simulink model "segway_torque_control"  (R2022a)
settings: Solver=FixedStepAuto  StartTime=0.0  StopTime=10  FixedStep=1e-3  RelTol=1e-3
PreLoadFcn:
  | preload
InitFcn:
  | init
  | preload
values from neighbouring files (symbols this model uses):
  A1 = [0 0   1 0 ... (first row only)    [plant.m]
  A2 = [0   1 ... (first row only)    [plant.m]
  alpha = n * Kt    [plant.m]
  B1 = [0 0 ... (first row only)    [plant.m]
  B2 = [0    0 ... (first row only)    [plant.m]
  C1 = [1 0 0 0 ... (first row only)    [plant.m]
  C2 = [1 0 ... (first row only)    [plant.m]
  chi0 = zeros(N_ukf, 2*N_ukf+1)    [UKF_params.m]
  D = 0.2    [params.m]
  D1 = zeros(4, 2)    [plant.m]
  D2 = zeros(2)    [plant.m]
  Fd = sysd.A    [LKF_params.m]
  fm = evalin('base', 'fm')    [f.m]    (also in params.m = 0.0022)
  fw = 0.0    (= 0)    [params.m]
  g = 9.81    [params.m]
  Gd = sysd.B    [LKF_params.m]
  h = 0.39    [params.m]
  H_ekf = [0 1 0 0 0 0 0 ... (first row only)    [EKF_params.m]
  H_lkf = [0 1 0 0 0 0 0 ... (first row only)    [LKF_params.m]
  H_ukf = [0 1 0 0 0 0 0 ... (first row only)    [UKF_params.m]
  Jm = 1e-5    (= 1e-05)    [params.m]
  Jphi = M * (W^2 + D^2) / 12    (= 0.126774333333)    [params.m]
  Jpsi = M * L^2 / 3    (= 0.08910525)    [params.m]
  Jw = m * R^2 / 2    (= 0.01146068)    [params.m]
  Jwx = m * (3*R^2 + hw^2) / 12    (= 0.00610456)    [params.m]
  K_lqr = lqrd(s4.A, s4.B, QQ, RR, Ts)    [control.m]
  Kt = 2.28    [params.m]
  L = h / 2    (= 0.195)    [params.m]
  lambda_ukf = alpha_ukf^2 * (N_ukf + kappa_ukf) - N_ukf    [UKF_params.m]
  M = 7.03    [params.m]
  m = 1.54    [params.m]
  n = 1    [params.m]
  N_ukf = length(x0_ukf)    [UKF_params.m]
  P0_ekf = eye(7)*0.1    [EKF_params.m]
  P0_lkf = eye(7)*0.1    [LKF_params.m]
  P0_ukf = eye(7)*0.1    [UKF_params.m]
  Q_ekf = [0.1*Ts^4/4     Ts^3/2     0          Ts^2/2     0          0          0 ... (first row only)    [EKF_params.m]
  Q_lkf = [Ts^4/4     Ts^3/2     0          Ts^2/2     0          0          0 ... (first row only)    [LKF_params.m]
  Q_ukf = [0.0025*Ts^4 Ts^3/2     0          Ts^2/2     0          0          0 ... (first row only)    [UKF_params.m]
  R = 0.122    [params.m]
  R_ekf = [sigma_y_ekf(1) 0          0          0          0 ... (first row only)    [EKF_params.m]
  R_lkf = [sigma_y(1) 0          0          0          0 ... (first row only)    [LKF_params.m]
  R_ukf = [sigma_y_ukf(1) 0          0          0          0 ... (first row only)    [UKF_params.m]
  Ts = 0.01    [params.m]
  W = 0.42    [params.m]
  w_c_ukf = diag(wi*ones([1, 2*N_ukf+1]))    [UKF_params.m]
  w_m_ukf = wi*ones([1, 2*N_ukf+1])    [UKF_params.m]
  x0_ekf = [0; 0; 0; 0; 0; 0; 0]    [EKF_params.m]
  x0_lkf = [0; 0; 0; 0; 0; 0; 0]    [LKF_params.m]
  x0_ukf = [0; 0; 0; 0; 0; 0; 0]    [UKF_params.m]
  Z0_ukf = zeros(5, 2*N_ukf+1)    [UKF_params.m]
undefined symbols (not defined in the file or in its folder): X, Y, Z
libraries: sm_lib x18, nesl_utility x14, simulink_extras x4, simulink x1
(part 1 of 2)
settings Model: Creator=skakd  LastModifiedBy=Yoggi
settings SolverCC: ZeroCrossControl=EnableAll  ZeroCrossAlgorithm=Adaptive  EnableFixedStepZeroCrossing=on

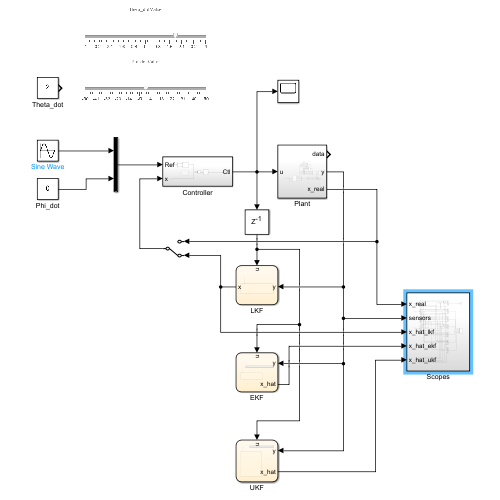
[thumbnail: Simulink's stored preview of the top-level diagram]
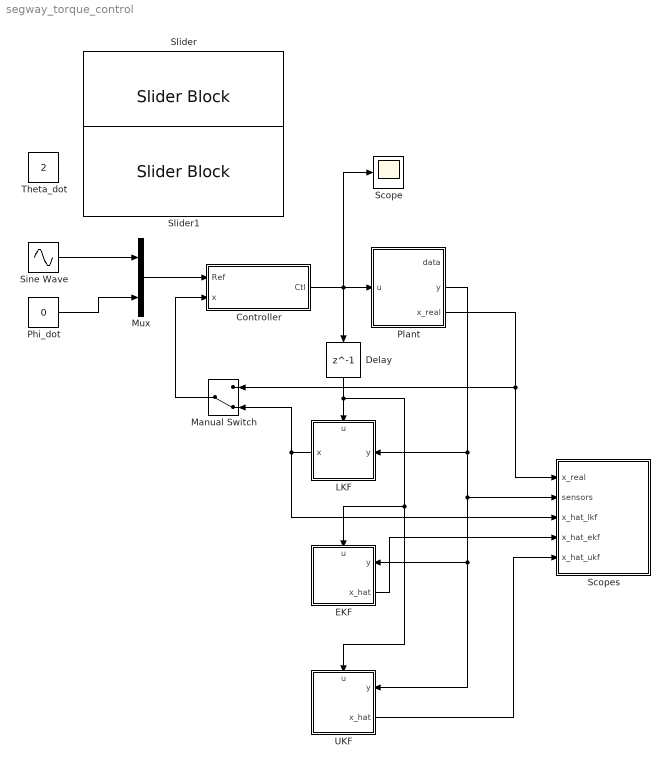
== system segway_torque_control ==
  Controller : Subsystem  SystemSampleTime=0.01
  Delay : Delay  DelayLength=1
  EKF : Stateflow chart  TreatAsAtomicUnit=on  SystemSampleTime=Ts
      settings: PortSchema="{\"entries\":[{\"content\":{\"sides\":[{\"content\":{\"connectorIds\":[]},\"type\":\"ConnectorPlacement.EquallySpacedRectSide\",\"uuid\":\"7365e1c5-a084-40ff-bf9b-f6bb3324d08a\"},{\"content\":{\"connectorIds\":[\"In2\",\"Out1\"],\"side\":\"RIGHT\"},\"type\":\"ConnectorPlacement.EquallySpacedRectSide\",\"uuid\":\"e745d55e-2f97-4317-b982-3a71d81393c6\"},{\"content\":{\"connectorIds\":[\"In1\"],\"side\":\"TOP\"},\"type\":\"ConnectorPlacement.EquallySpacedRectSide\",\"uuid\":\"33cc398c-7f08-41ce-89d7-3873ba12ad1e\"}]},\"type\":\"ConnectorPlacement.EquallySpacedConnector\",\"uuid\":\"9c830667-db1c-4875-b9da-b2b8107bc2bd\"}],\"packageUris\":[\"http://schema.mathworks.com/mf0/Connector/R2020b\"],\"version\":\"1.0\"}"
  LKF : Stateflow chart  TreatAsAtomicUnit=on  SystemSampleTime=Ts
      settings: PortSchema="{\"entries\":[{\"content\":{\"sides\":[{\"content\":{\"connectorIds\":[\"Out1\"]},\"type\":\"ConnectorPlacement.EquallySpacedRectSide\",\"uuid\":\"7365e1c5-a084-40ff-bf9b-f6bb3324d08a\"},{\"content\":{\"connectorIds\":[\"In2\"],\"side\":\"RIGHT\"},\"type\":\"ConnectorPlacement.EquallySpacedRectSide\",\"uuid\":\"e745d55e-2f97-4317-b982-3a71d81393c6\"},{\"content\":{\"connectorIds\":[\"In1\"],\"side\":\"TOP\"},\"type\":\"ConnectorPlacement.EquallySpacedRectSide\",\"uuid\":\"33cc398c-7f08-41ce-89d7-3873ba12ad1e\"}]},\"type\":\"ConnectorPlacement.EquallySpacedConnector\",\"uuid\":\"9c830667-db1c-4875-b9da-b2b8107bc2bd\"}],\"packageUris\":[\"http://schema.mathworks.com/mf0/Connector/R2020b\"],\"version\":\"1.0\"}"
  Manual Switch : ManualSwitch  CurrentSetting=0
  Mux : Mux  Inputs=2
  Phi_dot : Constant  Value=0
  Plant : Subsystem
  Scope : Scope
  Scopes : Subsystem
  Sine Wave : Sin  SampleTime=0
  Slider : SliderBlock  ScaleMin=-4  ScaleMax=4
  Slider1 : SliderBlock  ScaleMin=-50  ScaleMax=50
  Theta_dot : Constant  Value=2
  UKF : Stateflow chart  TreatAsAtomicUnit=on  SystemSampleTime=Ts
      settings: PortSchema="{\"entries\":[{\"content\":{\"sides\":[{\"content\":{\"connectorIds\":[]},\"type\":\"ConnectorPlacement.EquallySpacedRectSide\",\"uuid\":\"7365e1c5-a084-40ff-bf9b-f6bb3324d08a\"},{\"content\":{\"connectorIds\":[\"In2\",\"Out1\"],\"side\":\"RIGHT\"},\"type\":\"ConnectorPlacement.EquallySpacedRectSide\",\"uuid\":\"e745d55e-2f97-4317-b982-3a71d81393c6\"},{\"content\":{\"connectorIds\":[\"In1\"],\"side\":\"TOP\"},\"type\":\"ConnectorPlacement.EquallySpacedRectSide\",\"uuid\":\"33cc398c-7f08-41ce-89d7-3873ba12ad1e\"}]},\"type\":\"ConnectorPlacement.EquallySpacedConnector\",\"uuid\":\"9c830667-db1c-4875-b9da-b2b8107bc2bd\"}],\"packageUris\":[\"http://schema.mathworks.com/mf0/Connector/R2020b\"],\"version\":\"1.0\"}"
  wires:
  Phi_dot/1 -> Mux/2
  Mux/1 -> Controller/1(Ref)
  Controller/1(Ctl) -> Plant/1(u), Scope/1, Delay/1
  Plant/2(y) -> UKF/2(y), EKF/2(y), Scopes/2(sensors), LKF/2(y)
  Plant/3(x_real) -> Manual Switch/1, Scopes/1(x_real)
  Delay/1 -> EKF/1(u), UKF/1(u), LKF/1(u)
  LKF/1(x) -> Scopes/3(x_hat_lkf), Manual Switch/2
  Manual Switch/1 -> Controller/2(x)
  EKF/1(x_hat) -> Scopes/4(x_hat_ekf)
  Sine Wave/1 -> Mux/1
  UKF/1(x_hat) -> Scopes/5(x_hat_ukf)

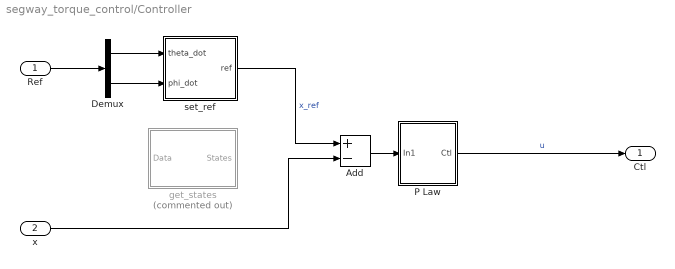
== system segway_torque_control/Controller ==
  Ref : Inport
  x : Inport  Port=2
  Add : Sum  Inputs=+-
  Demux : Demux  Outputs=2
  P Law : Subsystem  TreatAsAtomicUnit=on  SystemSampleTime=0.01
  get_states : Subsystem  Commented=on
  set_ref : Subsystem
  Ctl : Outport  VectorParamsAs1DForOutWhenUnconnected=off
  wires:
  P Law/1(Ctl) -> Ctl/1  "u"
  set_ref/1(ref) -> Add/1  "x_ref"
  Ref/1 -> Demux/1
  Demux/1 -> set_ref/1(theta_dot)
  Demux/2 -> set_ref/2(phi_dot)
  Add/1 -> P Law/1(In1)
  x/1 -> Add/2

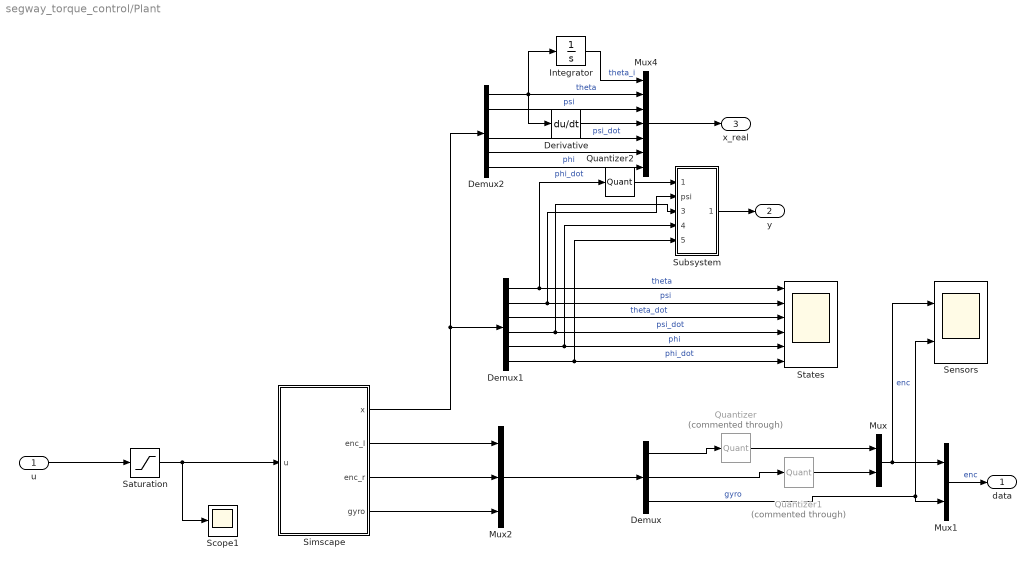
== system segway_torque_control/Plant ==
  u : Inport
  Demux : Demux  Outputs=3
  Demux1 : Demux  Outputs=6
  Demux2 : Demux  Outputs=6
  Derivative : Derivative
  Integrator : Integrator
  Mux : Mux  Inputs=2
  Mux1 : Mux  Inputs=2
  Mux2 : Mux  Inputs=3
  Mux4 : Mux  Inputs=7
  Quantizer : Quantizer  Commented=through  QuantizationInterval=pi/45
  Quantizer1 : Quantizer  Commented=through  QuantizationInterval=pi/45
  Quantizer2 : Quantizer  QuantizationInterval=pi/45
  Saturation : Saturate  UpperLimit=40  LowerLimit=-40
  Scope1 : Scope
  Sensors : Scope  NumInputPorts=2
  Simscape : Subsystem  Variant=on  VariantControl=Choice
  States : Scope  NumInputPorts=6
  Subsystem : Subsystem  TreatAsAtomicUnit=on  SystemSampleTime=Ts
  data : Outport
  y : Outport  Port=2
  x_real : Outport  Port=3
  wires:
  Mux2/1 -> Demux/1
  Demux/1 -> Quantizer/1
  Demux/2 -> Quantizer1/1
  Mux/1 -> Mux1/1, Sensors/1  "enc"
  Demux/3 -> Mux1/2, Sensors/2  "gyro"
  Demux1/3 -> States/3  "theta_dot"
  Demux1/1 -> States/1, Quantizer2/1  "theta"
  Demux1/4 -> Subsystem/3(psi_dot), States/4  "psi_dot"
  Demux1/6 -> Subsystem/5(phi_dot), States/6  "phi_dot"
  Demux1/2 -> Subsystem/2(psi), States/2  "psi"
  Demux1/5 -> Subsystem/4(phi), States/5  "phi"
  u/1 -> Saturation/1
  Saturation/1 -> Scope1/1, Simscape/1(u)
  Simscape/1(x) -> Demux2/1, Demux1/1
  Simscape/2(enc_l) -> Mux2/1
  Simscape/3(enc_r) -> Mux2/2
  Simscape/4(gyro) -> Mux2/3
  Mux1/1 -> data/1  "enc"
  Quantizer/1 -> Mux/1
  Quantizer1/1 -> Mux/2
  Demux2/1 -> Derivative/1, Mux4/2, Integrator/1  "theta"
  Integrator/1 -> Mux4/1  "theta_i"
  Demux2/2 -> Mux4/3  "psi"
  Demux2/4 -> Mux4/5  "psi_dot"
  Demux2/5 -> Mux4/6  "phi"
  Demux2/6 -> Mux4/7  "phi_dot"
  Mux4/1 -> x_real/1
  Derivative/1 -> Mux4/4
  Quantizer2/1 -> Subsystem/1(In1)
  Subsystem/1(Out1) -> y/1

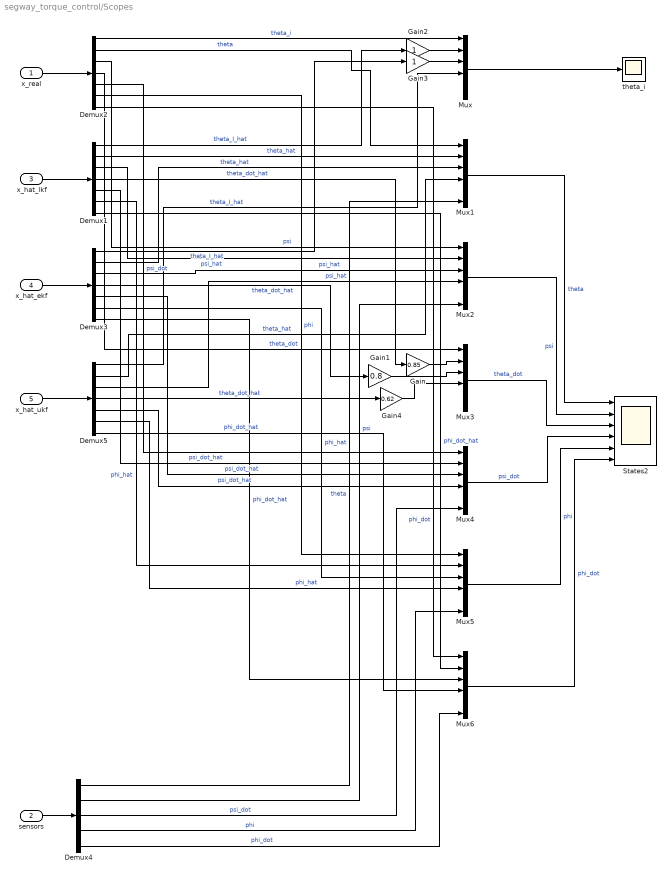
== system segway_torque_control/Scopes ==
  x_real : Inport
  sensors : Inport  Port=2
  x_hat_lkf : Inport  Port=3
  x_hat_ekf : Inport  Port=4
  x_hat_ukf : Inport  Port=5
  Demux{1..3,5} (4 alike) : Demux  Outputs=7
  Demux4 : Demux  Outputs=5
  Gain : Gain  Gain=0.85
  Gain1 : Gain  Gain=0.8
  Gain2 : Gain
  Gain3 : Gain
  Gain4 : Gain  Gain=0.62
  Mux{,1..6} (7 alike) : Mux  Inputs=6
  States2 : Scope  NumInputPorts=6
  theta_i : Scope
  wires:
  x_hat_lkf/1 -> Demux1/1
  x_real/1 -> Demux2/1
  Demux2/1 -> Mux/1  "theta_i"
  Demux1/1 -> Gain2/1  "theta_I_hat"
  Demux2/2 -> Mux1/1  "theta"
  Demux1/2 -> Mux1/2  "theta_hat"
  Demux2/3 -> Mux2/1  "psi"
  Demux2/4 -> Mux3/1  "theta_dot"
  Demux2/5 -> Mux4/1  "psi_dot"
  Demux2/6 -> Mux5/1  "phi"
  Demux2/7 -> Mux6/1  "phi_dot"
  Demux1/3 -> Mux2/2  "psi_hat"
  Demux1/4 -> Gain/1  "theta_dot_hat"
  Demux1/5 -> Mux4/2  "psi_dot_hat"
  Demux1/6 -> Mux5/2  "phi_hat"
  Demux1/7 -> Mux6/2  "phi_dot_hat"
  Mux1/1 -> States2/1  "theta"
  Mux2/1 -> States2/2  "psi"
  Mux3/1 -> States2/3  "theta_dot"
  Mux4/1 -> States2/4  "psi_dot"
  Mux5/1 -> States2/5  "phi"
  Mux6/1 -> States2/6  "phi_dot"
  Gain/1 -> Mux3/2
  x_hat_ekf/1 -> Demux3/1
  Mux/1 -> theta_i/1
  Demux3/1 -> Gain3/1  "theta_I_hat"
  Demux3/2 -> Mux1/3  "theta_hat"
  Demux3/3 -> Mux2/3  "psi_hat"
  Demux3/4 -> Gain1/1  "theta_dot_hat"
  Demux3/5 -> Mux4/3  "psi_dot_hat"
  Demux3/6 -> Mux5/3  "phi_hat"
  Demux3/7 -> Mux6/3  "phi_dot_hat"
  Gain1/1 -> Mux3/3
  Gain2/1 -> Mux/2
  Gain3/1 -> Mux/3
  sensors/1 -> Demux4/1
  Demux4/1 -> Mux1/6  "theta"
  Demux4/2 -> Mux2/6  "psi"
  Demux4/3 -> Mux4/6  "psi_dot"
  Demux4/4 -> Mux5/6  "phi"
  Demux4/5 -> Mux6/6  "phi_dot"
  x_hat_ukf/1 -> Demux5/1
  Demux5/1 -> Mux/4  "theta_I_hat"
  Demux5/2 -> Mux1/4  "theta_hat"
  Demux5/3 -> Mux2/4  "psi_hat"
  Demux5/4 -> Gain4/1  "theta_dot_hat"
  Demux5/5 -> Mux4/4  "psi_dot_hat"
  Demux5/6 -> Mux5/4  "phi_hat"
  Demux5/7 -> Mux6/4  "phi_dot_hat"
  Gain4/1 -> Mux3/4

== system segway_torque_control/Controller/P Law ==
  In1 : Inport
  Gain : Gain  Gain=K_lqr  Multiplication=Matrix(K*u)
  Ctl : Outport
  wires:
  Gain/1 -> Ctl/1
  In1/1 -> Gain/1

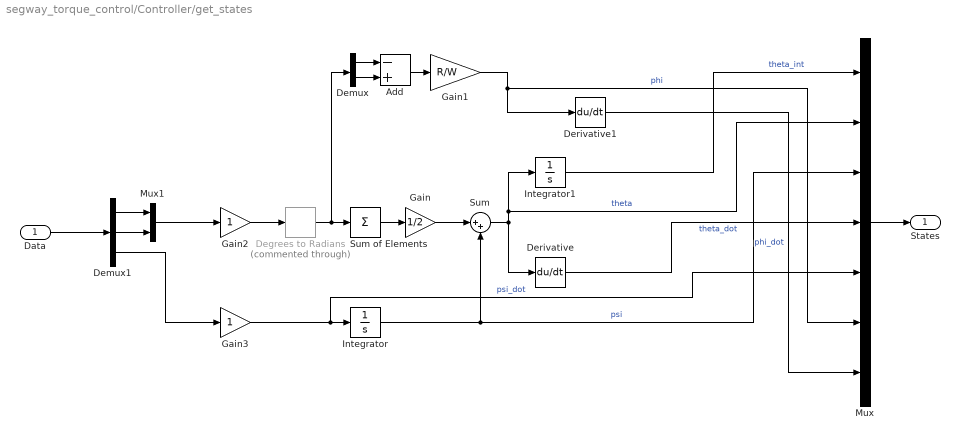
== system segway_torque_control/Controller/get_states ==
  Data : Inport
  Add : Sum  Inputs=-+
  Degrees to Radians : simulink_extras/Transformations/Degrees to Radians  Commented=through
  Demux : Demux  Outputs=2
  Demux1 : Demux  Outputs=3
  Derivative : Derivative
  Derivative1 : Derivative  CoefficientInTFapproximation=0.01
  Gain : Gain  Gain=1/2
  Gain1 : Gain  Gain=R/W
  Gain2 : Gain
  Gain3 : Gain
  Integrator : Integrator
  Integrator1 : Integrator
  Mux : Mux  Inputs=7
  Mux1 : Mux  Inputs=2
  Sum : Sum  Inputs=|++
  Sum of Elements : Sum  Inputs=+
  States : Outport  VectorParamsAs1DForOutWhenUnconnected=off
  wires:
  Gain/1 -> Sum/1
  Degrees to Radians/1 -> Demux/1, Sum of Elements/1
  Integrator/1 -> Sum/2, Mux/3  "psi"
  Data/1 -> Demux1/1
  Mux1/1 -> Gain2/1
  Sum/1 -> Mux/2, Integrator1/1, Derivative/1  "theta"
  Derivative/1 -> Mux/4  "theta_dot"
  Sum of Elements/1 -> Gain/1
  Gain3/1 -> Mux/5, Integrator/1  "psi_dot"
  Integrator1/1 -> Mux/1  "theta_int"
  Demux/1 -> Add/1
  Demux/2 -> Add/2
  Add/1 -> Gain1/1
  Gain1/1 -> Mux/6, Derivative1/1  "phi"
  Derivative1/1 -> Mux/7  "phi_dot"
  Mux/1 -> States/1
  Demux1/1 -> Mux1/1
  Demux1/2 -> Mux1/2
  Demux1/3 -> Gain3/1
  Gain2/1 -> Degrees to Radians/1

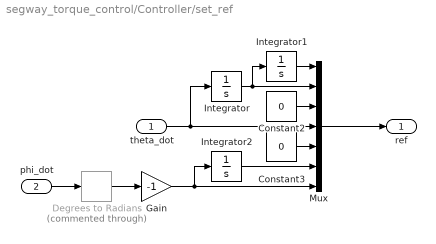
== system segway_torque_control/Controller/set_ref ==
  theta_dot : Inport
  phi_dot : Inport  Port=2
  Constant2 : Constant  Value=0
  Constant3 : Constant  Value=0
  Degrees to Radians : simulink_extras/Transformations/Degrees to Radians  Commented=through
  Gain : Gain  Gain=-1
  Integrator : Integrator
  Integrator1 : Integrator
  Integrator2 : Integrator
  Mux : Mux  Inputs=7
  ref : Outport  VectorParamsAs1DForOutWhenUnconnected=off
  wires:
  Constant2/1 -> Mux/3
  Constant3/1 -> Mux/5
  Mux/1 -> ref/1
  Integrator/1 -> Integrator1/1, Mux/2
  phi_dot/1 -> Degrees to Radians/1
  Integrator2/1 -> Mux/6
  Integrator1/1 -> Mux/1
  theta_dot/1 -> Integrator/1, Mux/4
  Degrees to Radians/1 -> Gain/1
  Gain/1 -> Integrator2/1, Mux/7

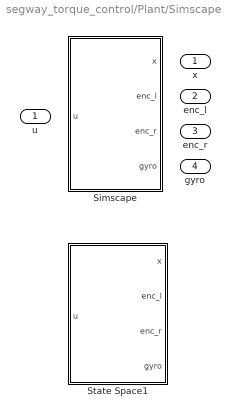
== system segway_torque_control/Plant/Simscape ==
  u : Inport
  Simscape : Subsystem  VariantControl=(default)
  State Space1 : Subsystem  VariantControl=is_simscape == 0
  x : Outport
  enc_l : Outport  Port=2
  enc_r : Outport  Port=3
  gyro : Outport  Port=4

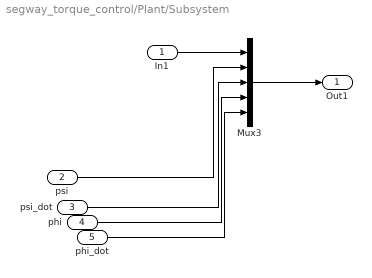
== system segway_torque_control/Plant/Subsystem ==
  In1 : Inport
  psi : Inport  Port=2
  psi_dot : Inport  Port=3
  phi : Inport  Port=4
  phi_dot : Inport  Port=5
  Mux3 : Mux  Inputs=5
  Out1 : Outport
  wires:
  In1/1 -> Mux3/1
  phi_dot/1 -> Mux3/5
  phi/1 -> Mux3/4
  Mux3/1 -> Out1/1
  psi_dot/1 -> Mux3/3
  psi/1 -> Mux3/2

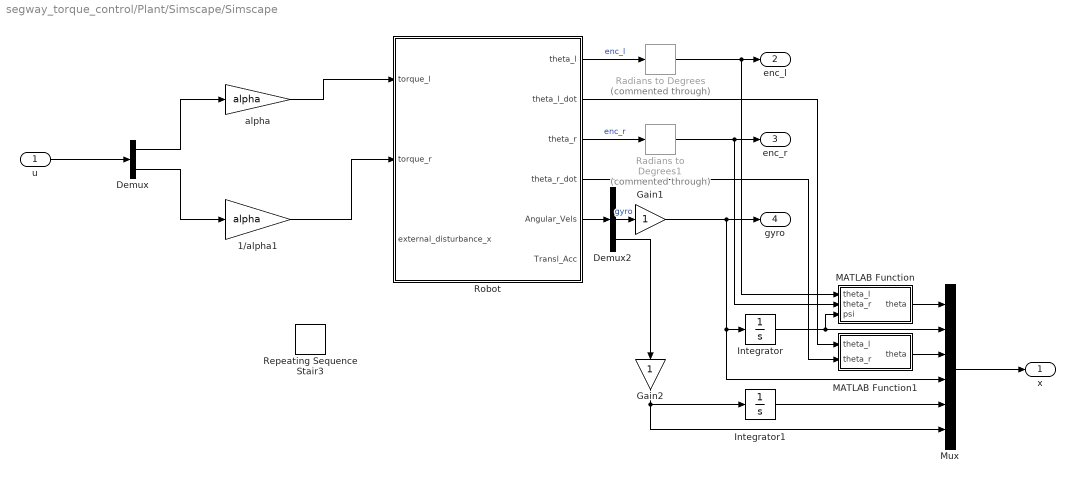
== system segway_torque_control/Plant/Simscape/Simscape ==
  u : Inport
  1/alpha1 : Gain  Gain=alpha
  Demux : Demux  Outputs=2
  Demux2 : Demux  Outputs=3
  Gain1 : Gain
  Gain2 : Gain
  Integrator : Integrator
  Integrator1 : Integrator
  MATLAB Function : MATLAB Function  TreatAsAtomicUnit=on
  MATLAB Function1 : MATLAB Function  TreatAsAtomicUnit=on
  Mux : Mux  Inputs=6
  Radians to Degrees : simulink_extras/Transformations/Radians to Degrees  Commented=through
  Radians to Degrees1 : simulink_extras/Transformations/Radians to Degrees  Commented=through
  Repeating Sequence Stair3 : simulink/Sources/Repeating Sequence Stair  OutValues=[0 0 0 0 0 0 0 0 0 0 0 0 15 0 0 0 0 0 0 0 0 0 0 0 0 0 0 0 0 0 0 0 0 0 0 0 0 0 0 0].'  tsamp=0.1  OutMin=[]  OutMax=[]  OutDataTypeStr=double  OutputDataTypeScalingMode=double  OutDataType=fixdt(0,8)  ConRadixGroup=Best Precision: Vector-wise  OutScaling=2^-12
  Robot : Subsystem
  alpha : Gain  Gain=alpha
  x : Outport
  enc_l : Outport  Port=2
  enc_r : Outport  Port=3
  gyro : Outport  Port=4
  wires:
  Robot/5(Angular_Vels) -> Demux2/1
  Demux2/2 -> Gain1/1  "gyro"
  Radians to Degrees1/1 -> MATLAB Function/2(theta_r), enc_r/1
  Robot/3(theta_r) -> Radians to Degrees1/1  "enc_r"
  Radians to Degrees/1 -> MATLAB Function/1(theta_l), enc_l/1
  Robot/1(theta_l) -> Radians to Degrees/1  "enc_l"
  Gain1/1 -> gyro/1, Mux/4, Integrator/1
  u/1 -> Demux/1
  Mux/1 -> x/1
  Integrator/1 -> MATLAB Function/3(psi), Mux/2
  Integrator1/1 -> Mux/5
  MATLAB Function/1(theta) -> Mux/1
  MATLAB Function1/1(theta) -> Mux/3
  Robot/2(theta_l_dot) -> MATLAB Function1/1(theta_l)
  Robot/4(theta_r_dot) -> MATLAB Function1/2(theta_r)
  Gain2/1 -> Integrator1/1, Mux/6
  Demux2/3 -> Gain2/1
  alpha/1 -> Robot/1(torque_l)
  1/alpha1/1 -> Robot/2(torque_r)
  Demux/1 -> alpha/1
  Demux/2 -> 1/alpha1/1

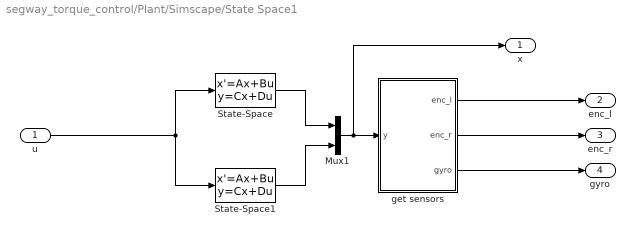
== system segway_torque_control/Plant/Simscape/State Space1 ==
  u : Inport
  Mux1 : Mux  Inputs=2
  State-Space : StateSpace  A=A1  B=B1  C=C1  D=D1  InitialCondition=0
  State-Space1 : StateSpace  A=A2  B=B2  C=C2  D=D2  InitialCondition=0
  get sensors : MATLAB Function  TreatAsAtomicUnit=on
  x : Outport
  enc_l : Outport  Port=2
  enc_r : Outport  Port=3
  gyro : Outport  Port=4
  wires:
  get sensors/3(gyro) -> gyro/1
  get sensors/2(enc_r) -> enc_r/1
  State-Space1/1 -> Mux1/2
  u/1 -> State-Space1/1, State-Space/1
  Mux1/1 -> get sensors/1(y), x/1
  State-Space/1 -> Mux1/1
  get sensors/1(enc_l) -> enc_l/1

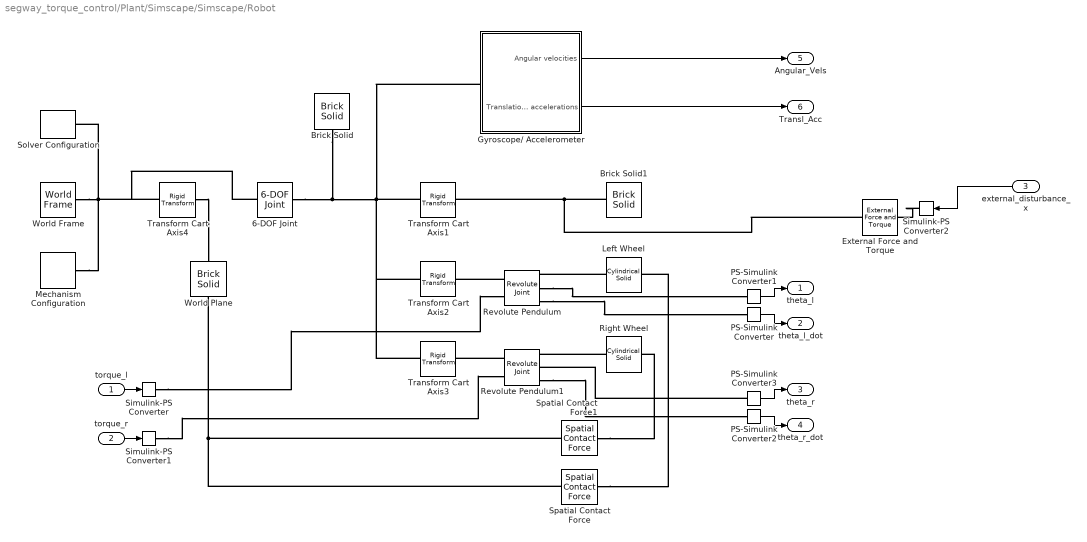
== system segway_torque_control/Plant/Simscape/Simscape/Robot ==
  torque_l : Inport
  torque_r : Inport  Port=2
  external_disturbance_x : Inport  Port=3
  6-DOF Joint : sm_lib/Joints/6-DOF Joint  JointMode=Normal  SenseConstraintForce=off  SenseConstraintForceX=off  SenseConstraintForceY=off  SenseConstraintForceZ=off  SenseConstraintTorque=off  SenseConstraintTorqueX=off  SenseConstraintTorqueY=off  SenseConstraintTorqueZ=off  SenseTotalForce=off  SenseTotalForceX=off  SenseTotalForceY=off  SenseTotalForceZ=off  SenseTotalTorque=off  SenseTotalTorqueX=off  SenseTotalTorqueY=off  SenseTotalTorqueZ=off  CompositeWrenchDir=FollowerOnBase  CompositeWrenchFrame=BaseFrame  PxEquilibriumPosition=0  PxEquilibriumPositionUnits=m  PxSpringStiffness=0  PxSpringStiffnessUnits=N/m  PxDampingCoefficient=0  PxDampingCoefficientUnits=N/(m/s)  PxTorqueActuationMode=NoTorque  PxMotionActuationMode=ComputedMotion  PxSensePosition=off  PxSenseVelocity=off  PxSenseAcceleration=off  PxSenseTorqueForce=off  PxSenseLowerLimitTorqueForce=off  PxSenseUpperLimitTorqueForce=off  PxLowerLimitSpecify=off  PxLowerLimitBound=-1  PxLowerLimitBoundUnits=m  PxLowerLimitStiffness=1e6  PxLowerLimitStiffnessUnits=N/m  PxLowerLimitDamping=1e3  PxLowerLimitDampingUnits=N/(m/s)  PxLowerLimitTransitionRegionWidth=1e-4  PxLowerLimitTransitionRegionWidthUnits=m  PxUpperLimitSpecify=off  PxUpperLimitBound=1  PxUpperLimitBoundUnits=m  PxUpperLimitStiffness=1e6  PxUpperLimitStiffnessUnits=N/m  PxUpperLimitDamping=1e3  PxUpperLimitDampingUnits=N/(m/s)  PxUpperLimitTransitionRegionWidth=1e-4  PxUpperLimitTransitionRegionWidthUnits=m  PxPositionTargetSpecify=off  PxPositionTargetPriority=High  PxPositionTargetValue=0  PxPositionTargetValueUnits=m  PxVelocityTargetSpecify=off  PxVelocityTargetPriority=High  PxVelocityTargetValue=0  PxVelocityTargetValueUnits=m/s  PyEquilibriumPosition=0  PyEquilibriumPositionUnits=m  PySpringStiffness=0  PySpringStiffnessUnits=N/m  PyDampingCoefficient=0  PyDampingCoefficientUnits=N/(m/s)  PyTorqueActuationMode=NoTorque  PyMotionActuationMode=ComputedMotion  PySensePosition=off  PySenseVelocity=off  PySenseAcceleration=off  PySenseTorqueForce=off  PySenseLowerLimitTorqueForce=off  PySenseUpperLimitTorqueForce=off  PyLowerLimitSpecify=off  PyLowerLimitBound=-1  PyLowerLimitBoundUnits=m  PyLowerLimitStiffness=1e6  PyLowerLimitStiffnessUnits=N/m  PyLowerLimitDamping=1e3  PyLowerLimitDampingUnits=N/(m/s)  PyLowerLimitTransitionRegionWidth=1e-4  PyLowerLimitTransitionRegionWidthUnits=m  PyUpperLimitSpecify=off  PyUpperLimitBound=1  PyUpperLimitBoundUnits=m  PyUpperLimitStiffness=1e6  PyUpperLimitStiffnessUnits=N/m  PyUpperLimitDamping=1e3  PyUpperLimitDampingUnits=N/(m/s)  PyUpperLimitTransitionRegionWidth=1e-4  PyUpperLimitTransitionRegionWidthUnits=m  PyPositionTargetSpecify=off  PyPositionTargetPriority=High  PyPositionTargetValue=0  PyPositionTargetValueUnits=m  PyVelocityTargetSpecify=off  PyVelocityTargetPriority=High  PyVelocityTargetValue=0  PyVelocityTargetValueUnits=m/s  PzEquilibriumPosition=0  PzEquilibriumPositionUnits=m  PzSpringStiffness=0  PzSpringStiffnessUnits=N/m  PzDampingCoefficient=0  PzDampingCoefficientUnits=N/(m/s)  PzTorqueActuationMode=NoTorque  PzMotionActuationMode=ComputedMotion  PzSensePosition=off  PzSenseVelocity=off  PzSenseAcceleration=off  PzSenseTorqueForce=off  PzSenseLowerLimitTorqueForce=off  PzSenseUpperLimitTorqueForce=off  PzLowerLimitSpecify=off  PzLowerLimitBound=-1  PzLowerLimitBoundUnits=m  PzLowerLimitStiffness=1e6  PzLowerLimitStiffnessUnits=N/m  PzLowerLimitDamping=1e3  PzLowerLimitDampingUnits=N/(m/s)  PzLowerLimitTransitionRegionWidth=1e-4  PzLowerLimitTransitionRegionWidthUnits=m  PzUpperLimitSpecify=off  PzUpperLimitBound=1  PzUpperLimitBoundUnits=m  PzUpperLimitStiffness=1e6  PzUpperLimitStiffnessUnits=N/m  PzUpperLimitDamping=1e3  PzUpperLimitDampingUnits=N/(m/s)  PzUpperLimitTransitionRegionWidth=1e-4  PzUpperLimitTransitionRegionWidthUnits=m  PzPositionTargetSpecify=on  PzPositionTargetPriority=High  PzPositionTargetValue=R+0.025  PzPositionTargetValueUnits=m  PzVelocityTargetSpecify=off  PzVelocityTargetPriority=High  PzVelocityTargetValue=0  PzVelocityTargetValueUnits=m/s  SphDefPosRotationMethod=None  SphDefPosRotationAngleUnits=deg  SphDefPosRotationStandardAxis=+Z  SphDefPosRotationAngle=0.0  SphDefPosRotationArbitraryAxis=[0 0 1]  SphDefPosFollAlignAxisA=+X  SphDefPosBaseAlignAxisA=+Y  SphDefPosFollAlignAxisB=+Y  SphDefPosBaseAlignAxisB=+Z  SphDefPosRotationSequenceAxes=FollowerAxes  SphDefPosRotationSequence=XYX  SphDefPosRotationSequenceAngles=[0 0 0]  SphDefPosRotationSequenceAnglesUnits=deg  SphDefPosRotationMatrix=[1 0 0; 0 1 0; 0 0 1]  SphEqPosRotationMethod=None  SphEqPosRotationAngleUnits=deg  SphEqPosRotationStandardAxis=+Z  SphEqPosRotationAngle=0.0  SphEqPosRotationArbitraryAxis=[0 0 1]  SphEqPosFollAlignAxisA=+X  SphEqPosBaseAlignAxisA=+Y  SphEqPosFollAlignAxisB=+Y  SphEqPosBaseAlignAxisB=+Z  SphEqPosRotationSequenceAxes=FollowerAxes  SphEqPosRotationSequence=XYX  SphEqPosRotationSequenceAngles=[0 0 0]  SphEqPosRotationSequenceAnglesUnits=deg  SphEqPosRotationMatrix=[1 0 0; 0 1 0; 0 0 1]  SphSpringStiffness=0  SphSpringStiffnessUnits=N*m/deg  SphDampingCoefficient=0  SphDampingCoefficientUnits=N*m/(deg/s)  SphActuateTorqueX=off  SphActuateTorqueY=off  SphActuateTorqueZ=off  SphActuateTorque=off  SphTorqueActuationMode=NoTorque  SphMotionActuationMode=ComputedMotion  SphActuationFrame=BaseFrame  SphSensePosition=off  SphSenseVelocityX=off  SphSenseVelocityY=off  SphSenseVelocityZ=off  SphSenseVelocity=off  SphSenseAccelerationX=off  SphSenseAccelerationY=off  SphSenseAccelerationZ=off  SphSenseAcceleration=off  SphSenseTorqueX=off  SphSenseTorqueY=off  SphSenseTorqueZ=off  SphSenseTorqueForce=off  SphSenseLowerLimitTorqueMag=off  SphSenseUpperLimitTorqueMag=off  SphSensingFrame=BaseFrame  SphLowerLimitSpecify=off  SphLowerLimitBound=15  SphLowerLimitBoundUnits=deg  SphLowerLimitStiffness=1e4  SphLowerLimitStiffnessUnits=N*m/deg  SphLowerLimitDamping=10  SphLowerLimitDampingUnits=N*m/(deg/s)  SphLowerLimitTransitionRegionWidth=0.1  SphLowerLimitTransitionRegionWidthUnits=deg  SphUpperLimitSpecify=off  SphUpperLimitBound=45  SphUpperLimitBoundUnits=deg  SphUpperLimitStiffness=1e4  SphUpperLimitStiffnessUnits=N*m/deg  SphUpperLimitDamping=10  SphUpperLimitDampingUnits=N*m/(deg/s)  SphUpperLimitTransitionRegionWidth=0.1  SphUpperLimitTransitionRegionWidthUnits=deg  SphPositionTargetRotationMethod=None  SphPositionTargetRotationAngleUnits=deg  SphPositionTargetRotationStandardAxis=+Z  SphPositionTargetRotationAngle=0.0  SphPositionTargetRotationArbitraryAxis=[0 0 1]  SphPositionTargetFollAlignAxisA=+X  SphPositionTargetBaseAlignAxisA=+Y  SphPositionTargetFollAlignAxisB=+Y  SphPositionTargetBaseAlignAxisB=+Z  SphPositionTargetRotationSequenceAxes=FollowerAxes  SphPositionTargetRotationSequence=XYX  SphPositionTargetRotationSequenceAngles=[0 0 0]  SphPositionTargetRotationSequenceAnglesUnits=deg  SphPositionTargetRotationMatrix=[1 0 0; 0 1 0; 0 0 1]  SphPositionTargetSpecify=off  SphPositionTargetPriority=High  SphVelocityTargetValue=[0 0 0]  SphVelocityTargetValueUnits=deg/s  SphVelocityTargetSpecify=off  SphVelocityTargetPriority=High  SphVelocityTargetInFollowerFrame=on
  Brick Solid : sm_lib/Body Elements/Brick Solid  GraphicAmbientColor=[0.15 0.15 0.15 1.0]  BasedOnType=Density  BrickDimensions=[0.01 W 0.01]  BrickDimensionUnits=m  CenterOfMass=[0 0 0]  CenterOfMassUnits=m  GraphicDiffuseColor=[0.5 0.5 0.5]  Density=10  DensityUnits=kg/m^3  DoExposeReferenceFrame=on  GraphicEmissiveColor=[0.0 0.0 0.0 1.0]  ExportEntireGeometry=off  SerializedFrames=<Frames/>  MarkerShape=Sphere  MarkerSize=10  GraphicType=FromGeometry  InertiaType=CalculateFromGeometry  Mass=10  MassUnits=kg  MomentsOfInertia=[1 1 1]  MomentsOfInertiaUnits=kg*m^2  GraphicOpacity=1.0  ProductsOfInertia=[0 0 0]  ProductsOfInertiaUnits=kg*m^2  GraphicShininess=75  GraphicSpecularColor=[0.5 0.5 0.5 1.0]  GraphicVisPropType=SimpleVisualProperties
  Brick Solid1 : sm_lib/Body Elements/Brick Solid  GraphicAmbientColor=[0.15 0.15 0.15 1.0]  BasedOnType=Mass  BrickDimensions=[D W h]  BrickDimensionUnits=m  CenterOfMass=[0 0 0]  CenterOfMassUnits=m  GraphicDiffuseColor=[1.0 1.0 0.0]  Density=40000  DensityUnits=kg/m^3  DoExposeReferenceFrame=on  GraphicEmissiveColor=[0.0 0.0 0.0 1.0]  ExportEntireGeometry=on  SerializedFrames=<Frames/>  MarkerShape=Sphere  MarkerSize=10  GraphicType=FromGeometry  InertiaType=CalculateFromGeometry  Mass=M  MassUnits=kg  MomentsOfInertia=[1 1 1]  MomentsOfInertiaUnits=kg*m^2  GraphicOpacity=1.0  ProductsOfInertia=[0 0 0]  ProductsOfInertiaUnits=kg*m^2  GraphicShininess=75  GraphicSpecularColor=[0.5 0.5 0.5 1.0]  GraphicVisPropType=SimpleVisualProperties
  External Force and Torque : sm_lib/Forces and Torques/External Force and Torque  ForceResolutionFrame=AttachedFrame  EnableForceX=on  EnableForceY=off  EnableForceZ=off  EnableForce=off  TorqueResolutionFrame=AttachedFrame  EnableTorqueX=off  EnableTorqueY=off  EnableTorqueZ=off  EnableTorque=off
  Gyroscope/ Accelerometer : Subsystem
  Left Wheel : sm_lib/Body Elements/Cylindrical Solid  GraphicAmbientColor=[0.15 0.15 0.15 1.0]  BasedOnType=Mass  CenterOfMass=[0 0 0]  CenterOfMassUnits=m  GraphicDiffuseColor=[0.2 0.2 0.2]  CylinderLength=hw  CylinderLengthUnits=m  CylinderRadius=R  CylinderRadiusUnits=m  Density=5000  DensityUnits=kg/m^3  DoExposeReferenceFrame=on  GraphicEmissiveColor=[0.0 0.0 0.0 1.0]  ExportEntireGeometry=on  SerializedFrames=<Frames/>  MarkerShape=Sphere  MarkerSize=10  GraphicType=FromGeometry  InertiaType=CalculateFromGeometry  Mass=m  MassUnits=kg  MomentsOfInertia=[0 0 Jw]  MomentsOfInertiaUnits=kg*m^2  GraphicOpacity=1.0  ProductsOfInertia=[0 0 0]  ProductsOfInertiaUnits=kg*m^2  GraphicShininess=75  GraphicSpecularColor=[0.5 0.5 0.5 1.0]  GraphicVisPropType=SimpleVisualProperties
  Mechanism Configuration : sm_lib/Utilities/Mechanism Configuration  UniformGravity=Constant  GravityVector=[0 0 -9.80665]  GravityUnits=m/s^2  LinearizationDelta=0.001  JointModeTransitionNonlinearIterations=2
  PS-Simulink Converter{,1..3} (4 alike) : nesl_utility/PS-Simulink Converter  PhysicalDomain=network_engine_domain  SubClassName=ps_output  LeftPortType=input  RightPortType=output  PseudoPeriodic=off  Frequencies=[]  VectorFormat=inherit  Unit=inherit  AffineConversion=off
      settings: SourceProductBaseCode=SS,PW,VE
  Revolute Pendulum : sm_lib/Joints/Revolute Joint  JointMode=Normal  SenseConstraintForce=off  SenseConstraintForceX=off  SenseConstraintForceY=off  SenseConstraintForceZ=off  SenseConstraintTorque=off  SenseConstraintTorqueX=off  SenseConstraintTorqueY=off  SenseConstraintTorqueZ=off  SenseTotalForce=off  SenseTotalForceX=off  SenseTotalForceY=off  SenseTotalForceZ=off  SenseTotalTorque=off  SenseTotalTorqueX=off  SenseTotalTorqueY=off  SenseTotalTorqueZ=off  CompositeWrenchDir=FollowerOnBase  CompositeWrenchFrame=BaseFrame  EquilibriumPosition=0  EquilibriumPositionUnits=deg  SpringStiffness=0  SpringStiffnessUnits=N*m/deg  DampingCoefficient=fm  DampingCoefficientUnits=N*m/(deg/s)  TorqueActuationMode=InputTorque  MotionActuationMode=ComputedMotion  SensePosition=on  SenseVelocity=on  SenseAcceleration=off  SenseTorqueForce=off  SenseLowerLimitTorqueForce=off  SenseUpperLimitTorqueForce=off  LowerLimitSpecify=off  LowerLimitBound=-90  LowerLimitBoundUnits=deg  LowerLimitStiffness=1e4  LowerLimitStiffnessUnits=N*m/deg  LowerLimitDamping=10  LowerLimitDampingUnits=N*m/(deg/s)  LowerLimitTransitionRegionWidth=0.1  LowerLimitTransitionRegionWidthUnits=deg  UpperLimitSpecify=off  UpperLimitBound=90  UpperLimitBoundUnits=deg  UpperLimitStiffness=1e4  UpperLimitStiffnessUnits=N*m/deg  UpperLimitDamping=10  UpperLimitDampingUnits=N*m/(deg/s)  UpperLimitTransitionRegionWidth=0.1  UpperLimitTransitionRegionWidthUnits=deg  PositionTargetSpecify=off  PositionTargetPriority=High  PositionTargetValue=0  PositionTargetValueUnits=deg  VelocityTargetSpecify=off  VelocityTargetPriority=High  VelocityTargetValue=0  VelocityTargetValueUnits=deg/s
  Revolute Pendulum1 : sm_lib/Joints/Revolute Joint  JointMode=Normal  SenseConstraintForce=off  SenseConstraintForceX=off  SenseConstraintForceY=off  SenseConstraintForceZ=off  SenseConstraintTorque=off  SenseConstraintTorqueX=off  SenseConstraintTorqueY=off  SenseConstraintTorqueZ=off  SenseTotalForce=off  SenseTotalForceX=off  SenseTotalForceY=off  SenseTotalForceZ=off  SenseTotalTorque=off  SenseTotalTorqueX=off  SenseTotalTorqueY=off  SenseTotalTorqueZ=off  CompositeWrenchDir=FollowerOnBase  CompositeWrenchFrame=BaseFrame  EquilibriumPosition=0  EquilibriumPositionUnits=deg  SpringStiffness=0  SpringStiffnessUnits=N*m/deg  DampingCoefficient=fm  DampingCoefficientUnits=N*m/(deg/s)  TorqueActuationMode=InputTorque  MotionActuationMode=ComputedMotion  SensePosition=on  SenseVelocity=on  SenseAcceleration=off  SenseTorqueForce=off  SenseLowerLimitTorqueForce=off  SenseUpperLimitTorqueForce=off  LowerLimitSpecify=off  LowerLimitBound=-90  LowerLimitBoundUnits=deg  LowerLimitStiffness=1e4  LowerLimitStiffnessUnits=N*m/deg  LowerLimitDamping=10  LowerLimitDampingUnits=N*m/(deg/s)  LowerLimitTransitionRegionWidth=0.1  LowerLimitTransitionRegionWidthUnits=deg  UpperLimitSpecify=off  UpperLimitBound=90  UpperLimitBoundUnits=deg  UpperLimitStiffness=1e4  UpperLimitStiffnessUnits=N*m/deg  UpperLimitDamping=10  UpperLimitDampingUnits=N*m/(deg/s)  UpperLimitTransitionRegionWidth=0.1  UpperLimitTransitionRegionWidthUnits=deg  PositionTargetSpecify=off  PositionTargetPriority=High  PositionTargetValue=0  PositionTargetValueUnits=deg  VelocityTargetSpecify=off  VelocityTargetPriority=High  VelocityTargetValue=0  VelocityTargetValueUnits=deg/s
  Right Wheel : sm_lib/Body Elements/Cylindrical Solid  GraphicAmbientColor=[0.15 0.15 0.15 1.0]  BasedOnType=Mass  CenterOfMass=[0 0 0]  CenterOfMassUnits=m  GraphicDiffuseColor=[0.2 0.2 0.2]  CylinderLength=hw  CylinderLengthUnits=m  CylinderRadius=R  CylinderRadiusUnits=m  Density=1000  DensityUnits=kg/m^3  DoExposeReferenceFrame=on  GraphicEmissiveColor=[0.0 0.0 0.0 1.0]  ExportEntireGeometry=on  SerializedFrames=<Frames/>  MarkerShape=Sphere  MarkerSize=10  GraphicType=FromGeometry  InertiaType=CalculateFromGeometry  Mass=m  MassUnits=kg  MomentsOfInertia=[Jwx Jwx Jw]  MomentsOfInertiaUnits=kg*m^2  GraphicOpacity=1.0  ProductsOfInertia=[0 0 0]  ProductsOfInertiaUnits=kg*m^2  GraphicShininess=75  GraphicSpecularColor=[0.5 0.5 0.5 1.0]  GraphicVisPropType=SimpleVisualProperties
  Simulink-PS Converter : nesl_utility/Simulink-PS Converter  PhysicalDomain=network_engine_domain  SubClassName=ps_input  LeftPortType=input  RightPortType=output  PseudoPeriodic=off  Frequencies=[]  NoiseDistribution=none  NoiseParameters=[]  Unit=1  AffineConversion=off  FilteringAndDerivatives=provide  SimscapeFilterOrder=1  InputFilterTimeConstant=0.001  UdotUserProvided=0
      settings: SourceProductBaseCode=SS,PW,VE
  Simulink-PS Converter1 : nesl_utility/Simulink-PS Converter  PhysicalDomain=network_engine_domain  SubClassName=ps_input  LeftPortType=input  RightPortType=output  PseudoPeriodic=off  Frequencies=[]  NoiseDistribution=none  NoiseParameters=[]  Unit=1  AffineConversion=off  FilteringAndDerivatives=provide  SimscapeFilterOrder=1  InputFilterTimeConstant=0.001  UdotUserProvided=0
      settings: SourceProductBaseCode=SS,PW,VE
  Simulink-PS Converter2 : nesl_utility/Simulink-PS Converter  PhysicalDomain=network_engine_domain  SubClassName=ps_input  LeftPortType=input  RightPortType=output  PseudoPeriodic=off  Frequencies=[]  NoiseDistribution=none  NoiseParameters=[]  Unit=1  AffineConversion=off  FilteringAndDerivatives=provide  SimscapeFilterOrder=1  InputFilterTimeConstant=0.001  UdotUserProvided=0
      settings: SourceProductBaseCode=SS,PW,VE
  Solver Configuration : nesl_utility/Solver Configuration  PhysicalDomain=network_engine_domain  SubClassName=solver  LeftPortType=input  RightPortType=generic  Tones=[]  Harmonics=[]  SimulateNoise=off  Profile=off  UseLocalSampling=off  EnableSwitchedLinearOptims=on  FrequencyDomain=off  UseCCode=off  RelTol=0.001  AbsTol=1e-06  MinStep=1e-09  ToWorkspace=off  RevertToSquareIcSolve=off  NumHomotopyIterations=100  PhasorMode=off  PhasorModeNumHarmonics=1  IndexReductionMethod=DerivativeReplacement  DoDC=off  ResidualTolerance=1e-09  UseLocalSolver=off  LocalSolverChoice=NE_BACKWARD_EULER_ADVANCER  LocalSolverSampleTime=0.001  DoFixedCost=off  MaxNonlinIter=3  MaxModeIter=2  ComputeImpulses=off  ImpulseIterations=2  LinearAlgebra=Sparse  LinearAlgebraNumThread=0  EquationFormulation=NE_TIME_EF  DelaysMemoryBudget=1024  AutomaticFiltering=on  FilteringTimeConstant=0.001  PartitionStorageMethod=AS_NEEDED  PartitionMemoryBudget=1024  PartitionMethod=FAST
      settings: SourceProductBaseCode=SS,PW,VE
  Spatial Contact Force : sm_lib/Forces and Torques/Spatial Contact Force  SenseContactBaseRotation=off  SenseContactBaseTranslation=off  CoefficientOfDynamicFriction=1  CoefficientOfStaticFriction=1  NormalDamping=1e3  NormalDampingUnits=N/(m/s)  SenseContactSignal=off  NormalStiffness=1e6  NormalStiffnessUnits=N/m  FrictionalCriticalVelocity=1e-2  FrictionalCriticalVelocityUnits=m/s  ZeroCrossDetectContactStartAndEnd=off  SenseContactFollowerRotation=off  SenseContactFollowerTranslation=off  FrictionType=SmoothStickSlip  SenseFrictionalForceMagnitude=off  SenseNormalForceMagnitude=off  NormalForceType=SmoothSpringDamper  SenseNormalVelocity=off  SenseSeparationDistance=off  SenseTangentialVelocity=off  NormalTransitionRegionWidth=1e-4  NormalTransitionRegionWidthUnits=m
  Spatial Contact Force1 : sm_lib/Forces and Torques/Spatial Contact Force  SenseContactBaseRotation=off  SenseContactBaseTranslation=off  CoefficientOfDynamicFriction=1  CoefficientOfStaticFriction=1  NormalDamping=1e3  NormalDampingUnits=N/(m/s)  SenseContactSignal=off  NormalStiffness=1e6  NormalStiffnessUnits=N/m  FrictionalCriticalVelocity=1e-2  FrictionalCriticalVelocityUnits=m/s  ZeroCrossDetectContactStartAndEnd=off  SenseContactFollowerRotation=off  SenseContactFollowerTranslation=off  FrictionType=SmoothStickSlip  SenseFrictionalForceMagnitude=off  SenseNormalForceMagnitude=off  NormalForceType=SmoothSpringDamper  SenseNormalVelocity=off  SenseSeparationDistance=off  SenseTangentialVelocity=off  NormalTransitionRegionWidth=1e-4  NormalTransitionRegionWidthUnits=m
  Transform Cart Axis1 : sm_lib/Frames and Transforms/Rigid Transform  TranslationMethod=StandardAxis  TranslationStandardOffset=L  TranslationLengthUnit=m  TranslationStandardAxis=+Z  TranslationCartesianOffset=[0 0 0]  TranslationROffset=0  TranslationROffsetUnits=m  TranslationZOffset=0  TranslationZOffsetUnits=m  TranslationThetaOffset=0  TranslationThetaOffsetUnits=deg  RotationMethod=None  RotationAngleUnits=deg  RotationStandardAxis=+Y  RotationAngle=90  RotationArbitraryAxis=[0 0 1]  FollAlignAxisA=+X  BaseAlignAxisA=+Y  FollAlignAxisB=+Y  BaseAlignAxisB=+Z  RotationSequenceAxes=FollowerAxes  RotationSequence=XYX  RotationSequenceAngles=[0 0 0]  RotationSequenceAnglesUnits=deg  RotationMatrix=[1 0 0; 0 1 0; 0 0 1]
  Transform Cart Axis2 : sm_lib/Frames and Transforms/Rigid Transform  TranslationMethod=StandardAxis  TranslationStandardOffset=W/2  TranslationLengthUnit=m  TranslationStandardAxis=+Y  TranslationCartesianOffset=[0 W/2 0]  TranslationROffset=0  TranslationROffsetUnits=m  TranslationZOffset=0  TranslationZOffsetUnits=m  TranslationThetaOffset=0  TranslationThetaOffsetUnits=deg  RotationMethod=StandardAxis  RotationAngleUnits=deg  RotationStandardAxis=+X  RotationAngle=90  RotationArbitraryAxis=[0 0 1]  FollAlignAxisA=+X  BaseAlignAxisA=+Y  FollAlignAxisB=+Y  BaseAlignAxisB=+Z  RotationSequenceAxes=FollowerAxes  RotationSequence=XYX  RotationSequenceAngles=[0 0 0]  RotationSequenceAnglesUnits=deg  RotationMatrix=[1 0 0; 0 1 0; 0 0 1]
  Transform Cart Axis3 : sm_lib/Frames and Transforms/Rigid Transform  TranslationMethod=StandardAxis  TranslationStandardOffset=W/2  TranslationLengthUnit=m  TranslationStandardAxis=-Y  TranslationCartesianOffset=[0 0 0]  TranslationROffset=0  TranslationROffsetUnits=m  TranslationZOffset=0  TranslationZOffsetUnits=m  TranslationThetaOffset=0  TranslationThetaOffsetUnits=deg  RotationMethod=RotationSequence  RotationAngleUnits=deg  RotationStandardAxis=+X  RotationAngle=90  RotationArbitraryAxis=[0 0 1]  FollAlignAxisA=+X  BaseAlignAxisA=+Y  FollAlignAxisB=+Y  BaseAlignAxisB=+Z  RotationSequenceAxes=FollowerAxes  RotationSequence=XYX  RotationSequenceAngles=[90 0 0]  RotationSequenceAnglesUnits=deg  RotationMatrix=[1 0 0; 0 1 0; 0 0 1]
  Transform Cart Axis4 : sm_lib/Frames and Transforms/Rigid Transform  TranslationMethod=StandardAxis  TranslationStandardOffset=0  TranslationLengthUnit=m  TranslationStandardAxis=+Z  TranslationCartesianOffset=[0 0 0]  TranslationROffset=0  TranslationROffsetUnits=m  TranslationZOffset=0  TranslationZOffsetUnits=m  TranslationThetaOffset=0  TranslationThetaOffsetUnits=deg  RotationMethod=StandardAxis  RotationAngleUnits=deg  RotationStandardAxis=+Y  RotationAngle=0  RotationArbitraryAxis=[0 0 1]  FollAlignAxisA=+X  BaseAlignAxisA=+Y  FollAlignAxisB=+Y  BaseAlignAxisB=+Z  RotationSequenceAxes=FollowerAxes  RotationSequence=XYX  RotationSequenceAngles=[0 0 0]  RotationSequenceAnglesUnits=deg  RotationMatrix=[1 0 0; 0 1 0; 0 0 1]
  World Frame : sm_lib/Frames and Transforms/World Frame
  World Plane : sm_lib/Body Elements/Brick Solid  GraphicAmbientColor=[0.15 0.15 0.15 1.0]  BasedOnType=Density  BrickDimensions=[100 100 0.05]  BrickDimensionUnits=m  CenterOfMass=[0 0 0]  CenterOfMassUnits=m  GraphicDiffuseColor=[0.0 0.8 0.0]  Density=1000  DensityUnits=kg/m^3  DoExposeReferenceFrame=on  GraphicEmissiveColor=[0.0 0.0 0.0 1.0]  ExportEntireGeometry=on  SerializedFrames=<Frames/>  MarkerShape=Sphere  MarkerSize=10  GraphicType=FromGeometry  InertiaType=PointMass  Mass=0.1  MassUnits=kg  MomentsOfInertia=[1 1 1]  MomentsOfInertiaUnits=kg*m^2  GraphicOpacity=1.0  ProductsOfInertia=[0 0 0]  ProductsOfInertiaUnits=kg*m^2  GraphicShininess=75  GraphicSpecularColor=[0.5 0.5 0.5 1.0]  GraphicVisPropType=SimpleVisualProperties
  theta_l : Outport
  theta_l_dot : Outport  Port=2
  theta_r : Outport  Port=3
  theta_r_dot : Outport  Port=4
  Angular_Vels : Outport  Port=5
  Transl_Acc : Outport  Port=6
  wires:
  torque_l/1 -> Simulink-PS Converter/1
  torque_r/1 -> Simulink-PS Converter1/1
  PS-Simulink Converter1/1 -> theta_l/1
  PS-Simulink Converter/1 -> theta_l_dot/1
  PS-Simulink Converter2/1 -> theta_r_dot/1
  PS-Simulink Converter3/1 -> theta_r/1
  Gyroscope/ Accelerometer/1(Angular velocities) -> Angular_Vels/1
  Gyroscope/ Accelerometer/2(Translation accelerations) -> Transl_Acc/1
  external_disturbance_x/1 -> Simulink-PS Converter2/1
  connections:
  Revolute Pendulum/RConn2 -- PS-Simulink Converter1/LConn1
  Spatial Contact Force1/RConn1 -- Right Wheel/LConn1
  Simulink-PS Converter1/RConn1 -- Revolute Pendulum1/LConn2
  Brick Solid1/RConn1 -- External Force and Torque/RConn1 -- Transform Cart Axis1/RConn1
  Spatial Contact Force/RConn1 -- Left Wheel/LConn1
  Revolute Pendulum1/LConn1 -- Transform Cart Axis3/RConn1
  Revolute Pendulum/LConn1 -- Transform Cart Axis2/RConn1
  6-DOF Joint/RConn1 -- Brick Solid/RConn1 -- Gyroscope/ Accelerometer/LConn1 -- Transform Cart Axis1/LConn1 -- Transform Cart Axis3/LConn1 -- Transform Cart Axis2/LConn1
  Transform Cart Axis4/RConn1 -- World Plane/RConn1
  Left Wheel/RConn1 -- Revolute Pendulum/RConn1
  Right Wheel/RConn1 -- Revolute Pendulum1/RConn1
  Spatial Contact Force1/LConn1 -- Spatial Contact Force/LConn1 -- World Plane/LConn1
  Mechanism Configuration/RConn1 -- Solver Configuration/RConn1 -- World Frame/RConn1 -- 6-DOF Joint/LConn1 -- Transform Cart Axis4/LConn1
  PS-Simulink Converter3/LConn1 -- Revolute Pendulum1/RConn2
  Revolute Pendulum1/RConn3 -- PS-Simulink Converter2/LConn1
  Simulink-PS Converter/RConn1 -- Revolute Pendulum/LConn2
  Revolute Pendulum/RConn3 -- PS-Simulink Converter/LConn1
  Simulink-PS Converter2/RConn1 -- External Force and Torque/LConn1

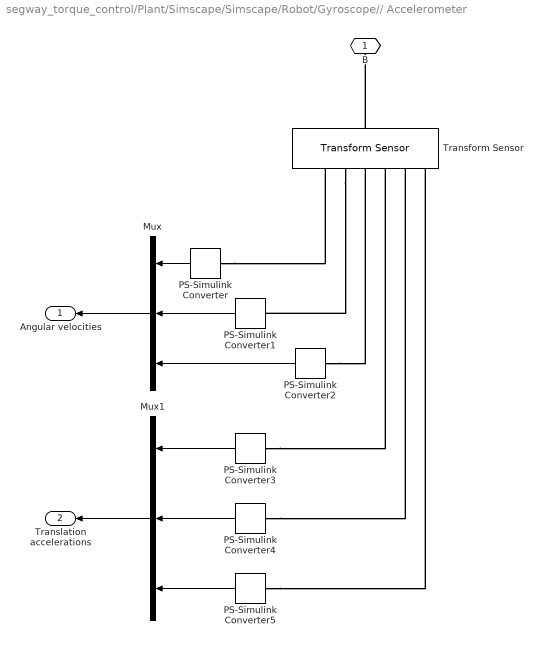
== system segway_torque_control/Plant/Simscape/Simscape/Robot/Gyroscope// Accelerometer ==
  Mux : Mux  Inputs=3
  Mux1 : Mux  Inputs=3
  PS-Simulink Converter{,1..5} (6 alike) : nesl_utility/PS-Simulink Converter  PhysicalDomain=network_engine_domain  SubClassName=ps_output  LeftPortType=input  RightPortType=output  PseudoPeriodic=off  Frequencies=[]  VectorFormat=1-D array  Unit=1  AffineConversion=off
      settings: SourceProductBaseCode=PW,SS
  Transform Sensor : sm_lib/Frames and Transforms/Transform Sensor  MeasurementFrame=Base  SenseAngle=off  SenseAxis=off  SenseAngle1=off  SenseAngle2=off  SenseAngle3=off  SenseQ=off  SenseR=off  SenseOmegaX=on  SenseOmegaY=on  SenseOmegaZ=on  SenseOmega1=off  SenseOmega2=off  SenseOmega3=off  SenseQDot=off  SenseRDot=off  SenseAlphaX=off  SenseAlphaY=off  SenseAlphaZ=off  SenseAlpha1=off  SenseAlpha2=off  SenseAlpha3=off  SenseQDDot=off  SenseRDDot=off  SenseX=off  SenseY=off  SenseZ=off  SenseRad=off  SenseAzim=off  SenseDist=off  SenseInc=off  SenseXDot=off  SenseYDot=off  SenseZDot=off  SenseRadDot=off  SenseAzimDot=off  SenseDistDot=off  SenseIncDot=off  SenseXDDot=on  SenseYDDot=on  SenseZDDot=on  SenseRadDDot=off  SenseAzimDDot=off  SenseDistDDot=off  SenseIncDDot=off
  B : PMIOPort  Side=Left
  Angular velocities : Outport
  Translation accelerations : Outport  Port=2
  wires:
  PS-Simulink Converter4/1 -> Mux1/2
  PS-Simulink Converter5/1 -> Mux1/3
  Mux/1 -> Angular velocities/1
  PS-Simulink Converter1/1 -> Mux/2
  PS-Simulink Converter2/1 -> Mux/3
  PS-Simulink Converter3/1 -> Mux1/1
  Mux1/1 -> Translation accelerations/1
  PS-Simulink Converter/1 -> Mux/1
  connections:
  PS-Simulink Converter4/LConn1 -- Transform Sensor/RConn6
  Transform Sensor/RConn3 -- PS-Simulink Converter1/LConn1
  PS-Simulink Converter5/LConn1 -- Transform Sensor/RConn7
  PS-Simulink Converter2/LConn1 -- Transform Sensor/RConn4
  PS-Simulink Converter3/LConn1 -- Transform Sensor/RConn5
  Transform Sensor/LConn1 -- B/RConn1
  PS-Simulink Converter/LConn1 -- Transform Sensor/RConn2

== matlab function segway_torque_control/Plant/Simscape/Simscape/MATLAB Function ==
  data: theta_l input; theta output; theta_r input; psi input
function theta = fcn(theta_l, theta_r, psi)

theta = (theta_l + theta_r)/2 + psi;

== stateflow chart segway_torque_control/LKF ==
  state Predict
    x_ = Fd * x + Gd * u;
    P_ = Fd * P * (Fd.') + Q_lkf;
    K_lkf = P_ * H_lkf.' * inv(H_lkf * P_*(H_lkf.') + R_lkf);
    x = x_ + K_lkf * (y - H_lkf * x_);
    P = (eye(7) - K_lkf * H_lkf) * P_ * ((eye(7) - K_lkf * H_lkf).') + K_lkf * R_lkf * (K_lkf.');
  (default) -> Predict : {x = x0_lkf; P = P0_lkf;}
  data: Fd parameter; Gd parameter; H_lkf parameter; P0_lkf parameter; u input; x0_lkf parameter; y input; P local; P_ local; x_ local; Q_lkf parameter; R_lkf parameter; x output; K_lkf local

== matlab function segway_torque_control/Plant/Simscape/Simscape/MATLAB Function1 ==
  data: theta_l input; theta output; theta_r input
function theta = fcn(theta_l, theta_r)

theta = (theta_l + theta_r)/2;

== stateflow chart segway_torque_control/EKF ==
  state Predict
    %PREDICT
    [x_, dfdx] = dynamics(x_hat, u, n ,fm, Kt, fw, m, M, L, R, W, Ts, Jm, Jw, Jpsi, Jphi, g);
    P_ = dfdx * P * (dfdx.') + Q_ekf;
    %UPDATE
    K_ekf = P_ * H_ekf.' * inv(H_ekf * P_*(H_ekf.') + R_ekf);
    x_hat = x_ + K_ekf * (y - H_ekf * x_);
    P = (eye(7) - K_ekf * H_ekf) * P_ * ((eye(7) - K_ekf * H_ekf).') + K_ekf * R_ekf * (K_ekf.');
  (default) -> Predict : {x_hat = x0_ekf; P = P0_ekf;}
  data: x function_input; u_ function_input; state function_output; n_ function_input; fm_ function_input; Kt_ function_input; fw_ function_input; m_ function_input; M_ function_input; L_ function_input; R_ function_input; W_ function_input; Ts_ function_input; Jm_ function_input; Jw_ function_input; Jpsi_ function_input; Jphi_ function_input; g_ function_input; jacobian function_output; u input; y input; P local; P_ local; x_ local; H_ekf parameter; Q_ekf parameter; R_ekf parameter; K_ekf local; dfdx local; P0_ekf parameter; fm parameter; n parameter; Kt parameter; Ts parameter; fw parameter; m parameter; L parameter; M parameter; R parameter; W parameter; x_hat output; Jm parameter; Jpsi parameter; Jw parameter; g parameter; Jphi parameter; x0_ekf parameter
  function [state, jacobian] = dynamics(x, u_, n_, fm_, Kt_, fw_, m_, M_, L_, R_, W_, Ts_, Jm_, Jw_, Jpsi_, Jphi_, g_):
    | 
    | function [state, jacobian] = dynamics(x, u_, n_, fm_, Kt_, fw_, m_, M_, L_, R_, W_, Ts_, Jm_, Jw_, Jpsi_, Jphi_, g_)
    |     alpha = n_*Kt_;
    |     beta = fm_;
    | 
    |     F_11 = 2*(beta+fw_);
    |     F_12 = -beta;
    |     F_21 = -beta;
    |     F_22 = beta;
    | 
    |     E_11 = (2*m_+M_)*R_^2 + 2*Jw_ + 2*n_^2*Jm_;
    |     E_12 = M_*L_*R_ - 2*n_^2*Jm_;
    |     E_21 = E_12;
    |     E_22 = M_*L_^2 + Jpsi_ + 2*n_^2*Jm_;
    |     detE = E_11*E_22 - E_12*E_21;
    | 
    |     I = 0.5*m_*W_^2 + Jphi_ + (W_^2/(2*R_^2))*(Jw_ + n_^2*Jm_);
    |     J = (W_^2/(2*R_^2))*(beta + fw_);
    |     K = (W_/(2*R_))*alpha;
    |     
    | 
    |     eq4 = -E_12*(-F_21*x(4) - F_22*x(5) + L_^2*M_*x(7)^2*sin(x(3))*cos(x(3)) + L_*M_*g_*sin(x(3)) + alpha*(-u_(1) - u_(2)))/detE + E_22*(-F_11*x(4) - F_12*x(5) + L_*M_*R_*x(5)^2*sin(x(3)) + alpha*(u_(1) + u_(2)))/detE;
    |     eq5 = E_11*(-F_21*x(4) - F_22*x(5) + L_^2*M_*x(7)^2*sin(x(3))*cos(x(3)) + L_*M_*g_*sin(x(3)) + alpha*(-u_(1) - u_(2)))/detE - E_21*(-F_11*x(4) - F_12*x(5) + L_*M_*R_*x(5)^2*sin(x(3)) + alpha*(u_(1) + u_(2)))/detE;
    |     eq6 = (-J*x(7) + K*(-u_(1) + u_(2)) - 2*L_^2*M_*x(5)*x(7)*sin(x(3))*cos(x(3)))/I;
    | 
    |     state = [x(1) + x(2)*Ts_; 
    |           x(2) + x(4)*Ts_; 
    |           x(3) + x(5)*Ts_; 
    |           x(4) + eq4*Ts_; 
    |           x(5) + eq5*Ts_; 
    |           x(6) + x(7)*Ts_; 
    |           x(7) + eq6*Ts_];
    | %     state = [alpha, beta, F_11, 4, 5, 6, 7];
    | 
    |     jacobian = eye(7);
    | 
    |     jacobian(1,2) = Ts_;
    |     jacobian(2,4) = Ts_;
    |     jacobian(3,5) = Ts_;
    |     jacobian(6,7) = Ts_;
    |     
    |     
    |     jacobian(4,3) = -Ts_*L_*M_*(E_12*(-2*L_*state(7)^2*sin(state(3))^2 + L_*state(7)^2 + g*cos(state(3))) - E_22*R*state(5)^2*cos(state(3)))/detE;
    |     jacobian(4,4) = (Ts_*(E_12*F_21 - E_22*F_11) + detE)/detE;
    |     jacobian(4,5) = Ts_*(E_12*F_22 - E_22*(F_12 - 2*L_*M_*R*state(5)*sin(state(3))))/detE;
    |     jacobian(4,7) = -Ts_*E_12*L_^2*M_*state(7)*sin(2*state(3))/detE;
    |     jacobian(5,3) = Ts_*L_*M_*(E_11*(-2*L_*state(7)^2*sin(state(3))^2 + L_*state(7)^2 + g*cos(state(3))) - E_21*R*state(5)^2*cos(state(3)))/detE;
    |     jacobian(5,4) = Ts_*(-E_11*F_21 + E_21*F_11)/detE;
    |     jacobian(5,5) = (-Ts_*(E_11*F_22 - E_21*(F_12 - 2*L_*M_*R*state(5)*sin(state(3)))) + detE)/detE;
    |     jacobian(5,7) = Ts_*E_11*L_^2*M_*state(7)*sin(2*state(3))/detE;
    | 
    |     jacobian(7,3) = -2*Ts_*L_^2*M_*state(5)*state(7)*cos(2*state(3))/I;
    |     jacobian(7,5) = -Ts_*L_^2*M_*state(7)*sin(2*state(3))/I;
    |     jacobian(7,7) = (-Ts_*(J + L_^2*M_*state(5)*sin(2*state(3))) + I)/I;
    | 
    | 
    | 
    | 
    | end

== matlab function segway_torque_control/Plant/Simscape/State Space1/get sensors ==
  data: enc_l output; enc_r output; y input; gyro output; R parameter; W parameter
function [enc_l, enc_r, gyro] = sensors(y, R, W)
enc_l = rad2deg(y(1) - W/R/2 * y(5) - y(2));
enc_r = rad2deg(y(1) + W/R/2 * y(5) - y(2));
gyro  = rad2deg(y(4));
